simulink library "Vehicle_Control_Axle2_Simple"  (R2024a)
settings: Solver=VariableStepAuto  StartTime=0.0  StopTime=10.0  RelTol=1e-3
libraries: Vehicle_Inputs x2, Brake_Control x1, Driveline_Control_Axle2_None x1, Power_Control_Axle2_FixedRatio x1
Description:
  | Simscape Vehicle Templates Library
  | 
  | Copyright 2018-2024 The MathWorks, Inc.
settings Model: Creator=smiller  LastModifiedBy=smiller
settings OptimizationCC: ReuseModelBlockBuffer=off
settings ModelReferenceCC: EnableRefExpFcnMdlSchedulingChecks=on
settings RTWCC: GPUComputeCapability=3.5

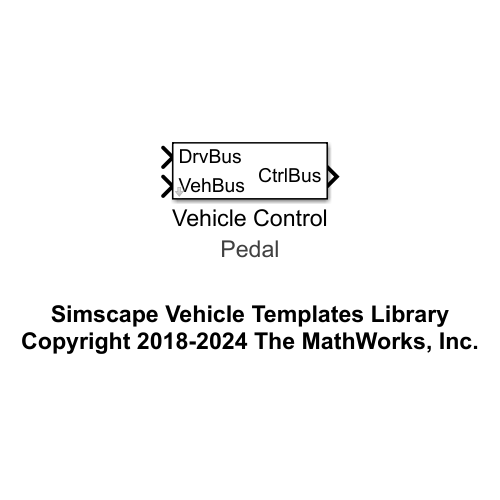
[thumbnail: Simulink's stored preview of the top-level diagram]
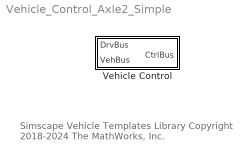
== system Vehicle_Control_Axle2_Simple ==
  note: Simscape Vehicle Templates Library
      | Copyright 2018-2024 The MathWorks, Inc.
  Vehicle Control : Subsystem  mask{popup_brake_control=Pedal, trq_ratio_front=1}
      mask prompts: popup_brake_control "Brake Control"; trq_ratio_front "Ratio of Torque on Front Wheels (0-1)"
      mask init:
      | if(popup_brake_control == 1)
      |     set_param([gcb '/Brake Control'],'popup_brake_control','Pedal');
      | elseif(popup_brake_control == 2)
      |     set_param([gcb '/Brake Control'],'popup_brake_control','Pressure');
      | elseif(popup_brake_control == 3)
      |     set_param([gcb '/Brake Control'],'popup_brake_control','ABS');
      | end
      settings: AttributesFormatString=%<popup_brake_control>
      mask TypeOptions popup_brake_control: Pedal | Pressure | ABS
      mask TypeOptions trq_ratio_front: Power Control/trq_ratio_front

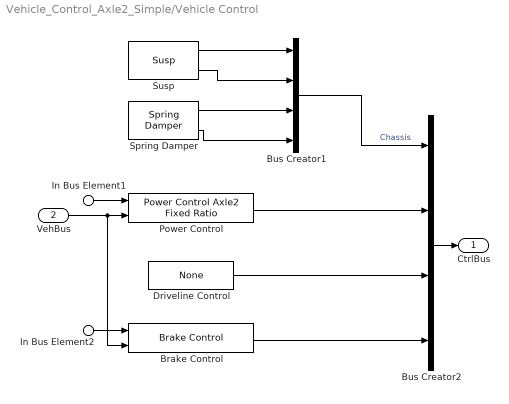
== system Vehicle_Control_Axle2_Simple/Vehicle Control ==
  In Bus Element1 : Inport  PortName=DrvBus  Element=rAccelPedal
  In Bus Element2 : Inport  PortName=DrvBus  Element=rBrakePedal
  VehBus : Inport  Port=2
  Brake Control : Brake_Control/Brake Control  VariantControl=Variant1  LabelModeActiveChoice=Pedal  popup_brake_control=Pedal  abs_tire_radiusF=0.35  abs_tire_radiusR=0.35
      settings: AttributesFormatString=%<ActiveVariant>
  Bus Creator1 : BusCreator  Inputs=4
  Bus Creator2 : BusCreator  Inputs=4
  Driveline Control : Driveline_Control_Axle2_None/None  SystemSampleTime=-1  VariantActivationTime=update diagram  AllowFlexibleInterface=on  Latency=0  AutoFrameSizeCalculation=off
  Power Control : Power_Control_Axle2_FixedRatio/Power Control Axle2 Fixed Ratio  trq_max=1600  trq_ratio_front=trq_ratio_front  trq_rate_up=300  trq_rate_down=-5000
  Spring Damper : Vehicle_Inputs/Control Bus/Spring Damper  SystemSampleTime=-1  VariantActivationTime=update diagram  AllowFlexibleInterface=on  Latency=0  AutoFrameSizeCalculation=off
  Susp : Vehicle_Inputs/Control Bus/Susp  SystemSampleTime=-1  VariantActivationTime=update diagram  AllowFlexibleInterface=on  Latency=0  AutoFrameSizeCalculation=off
  CtrlBus : Outport  VectorParamsAs1DForOutWhenUnconnected=off
  wires:
  Driveline Control/1 -> Bus Creator2/3
  Bus Creator2/1 -> CtrlBus/1
  Bus Creator1/1 -> Bus Creator2/1  "Chassis"
  VehBus/1 -> Power Control/2, Brake Control/2
  Brake Control/1 -> Bus Creator2/4
  Power Control/1 -> Bus Creator2/2
  In Bus Element2/1 -> Brake Control/1
  In Bus Element1/1 -> Power Control/1
  Susp/1 -> Bus Creator1/1
  Spring Damper/2 -> Bus Creator1/4
  Spring Damper/1 -> Bus Creator1/3
  Susp/2 -> Bus Creator1/2
